simulink model "kinctrltetis2"  (Simulink 8.1)
settings: Solver=ode45  StartTime=0.0  StopTime=10  FixedStep=0.03  MaxStep=0.1  RelTol=1e-4
values from neighbouring files (symbols this model uses):
  qr = [0 -pi/4 pi/2 -pi/4 ]    [mdl_tetis2.m]
libraries: roblocks x5, simulink x1
settings Model: Creator=fernando  LastModifiedBy=fernando

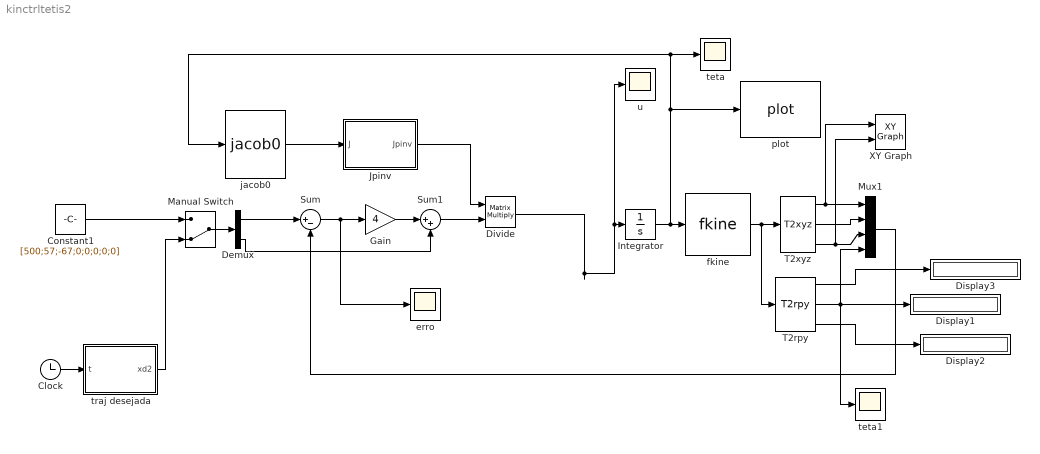
== system kinctrltetis2 ==
  Clock : Clock
  Constant1 : Constant  Value=[500;57;-67;0;0;0;0;0]
  Demux : Demux  Outputs=2
  Display1 : Display
  Display2 : Display
  Display3 : Display
  Divide : Product  Inputs=**  Multiplication=Matrix(*)
  Gain : Gain  Gain=4
  Integrator : Integrator  InitialCondition=qr+[0 0 0 0.1]  ZeroCross=off
  Jpinv : MATLAB Function  TreatAsAtomicUnit=on
  Manual Switch : ManualSwitch  CurrentSetting=0
  Mux1 : Mux
  Sum : Sum  Inputs=|+-
  Sum1 : Sum  Inputs=|++
  T2rpy : roblocks/Transform Conversion/T2rpy
  T2xyz : roblocks/Transform Conversion/T2xyz
  XY Graph : simulink/Sinks/XY Graph  xmin=-0  xmax=800  ymin=-300  ymax=100  st=-1
  erro : Scope
      settings: ShowLegends=on  TimeRange=9.99  YMin=-60  YMax=140  SaveName=ScopeData2
  fkine : roblocks/Kinematics/fkine  robot=Tetis
  "jacob0 " : roblocks/Kinematics/jacob0   robot=Tetis
  plot : roblocks/Robot Graphics/plot  robot=Tetis  fps=20  holdplot=on
  teta : Scope
      settings: TimeRange=10  YMin=-1.5  YMax=2.5
  teta1 : Scope
      settings: TimeRange=10  YMin=-0.32  YMax=-0.12  SaveName=ScopeData3
  traj desejada : MATLAB Function  TreatAsAtomicUnit=on
  u : Scope
      settings: YMin=-2.75  YMax=1.5
  wires:
  Integrator/1 -> plot/1, teta/1, "jacob0 "/1, fkine/1
  Jpinv/1(Jpinv) -> Divide/1
  Sum/1 -> Gain/1, erro/1
  fkine/1 -> T2rpy/1, T2xyz/1
  T2xyz/1 -> Mux1/1, XY Graph/1
  T2xyz/2 -> Mux1/2
  T2xyz/3 -> Mux1/3, XY Graph/2
  Mux1/1 -> Sum/2
  "jacob0 "/1 -> Jpinv/1(J)
  Constant1/1 -> Manual Switch/1
  Clock/1 -> traj desejada/1(t)
  traj desejada/1(xd2) -> Manual Switch/2
  Manual Switch/1 -> Demux/1
  Demux/1 -> Sum/1
  Sum1/1 -> Divide/2
  T2rpy/2 -> teta1/1, Mux1/4, Display1/1
  T2rpy/3 -> Display2/1
  T2rpy/1 -> Display3/1
  Demux/2 -> Sum1/2
  Gain/1 -> Sum1/1
  Divide/1 -> u/1, Integrator/1

== matlab function Jpinv ==
  data: J input double; Jpinv output double
function Jpinv = fcn(J)
%#codegen

Ja=[J(1:3,:);0 -1 -1 -1]; %;J(6,:)];
Jpinv = inv(Ja);

== matlab function traj desejada ==
  data: t input double; xd2 output double
function xd2  = fcn(t)
%#codegen

wn=2*pi/10;

%xd= [(200) 0 (250)]';
%xddot= [0 0 0]';
%xd= [(75*sin(wn*t)+500) 57 (75*cos(wn*t)-67) 0]';
%xddot= [75*wn*cos(wn*t) 0 -75*wn*sin(wn*t) 0]';

xd= [(75*(sin(wn*t)+sin(4*wn*t))+500) 57 (75*(cos(wn*t)+cos(4*wn*t))-67) pi/10*sin(wn*t)]';
xddot= [75*(wn*cos(wn*t)+4*wn*cos(4*wn*t)) 0 -75*(wn*sin(wn*t)+4*wn*sin(4*wn*t)) pi/10*wn*cos(wn*t)]';

xd2=[xd;xddot];
